simulink library "libGainScheduleDataLoader"  (R2020b)
settings: Solver=VariableStepAuto  StartTime=0.0  StopTime=10.0  RelTol=1e-3
undefined symbols (not defined in the file): range, scheduleData
settings Model: Creator=caatay  LastModifiedBy=caatay

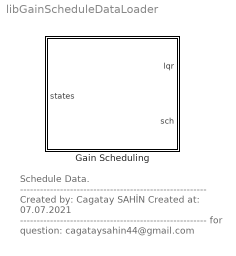
== system libGainScheduleDataLoader ==
  note: Schedule Data.
      | --------------------------------------------------------
      | Created by: Cagatay SAHİN
      | Created at: 07.07.2021
      | --------------------------------------------------------
      | for question:
      | cagataysahin44@gmail.com
  Gain Scheduling : Subsystem  mask(Flight Control System - Gain Scheduling Model - Scheduled Data Loader){scheduleData=scheduleData, range=range}
      mask prompts: scheduleData "Scheduling Data For FCS"; range "Scheduling Data Range"
      mask help: Aircraft's Stability Augmented System's schedule and gain data loader model.
      mask Help:
      | This block is used for obtain schedule database for stability augmented system to stabilize aircraft.
      | --------------------------------------------------------------------------------------------------------------------------------------------------
      | Input of the function:
      | 	states: State Information.
      | Output of the function:
      | 	K_{lqr}: LQR Gain Parameters.
      | 	sch: Scheduled Database Parameters.
      | --------------------------------------------------------------------------------------------------------------------------------------------------
      | for question: "cagataysahin44@gmail.com"
      mask Display:
      | port_label('input',1,'states','texmode','on');
      | 
      | port_label('output',1,'K_{lqr}','texmode','on');
      | port_label('output',2,'Sch','texmode','on');

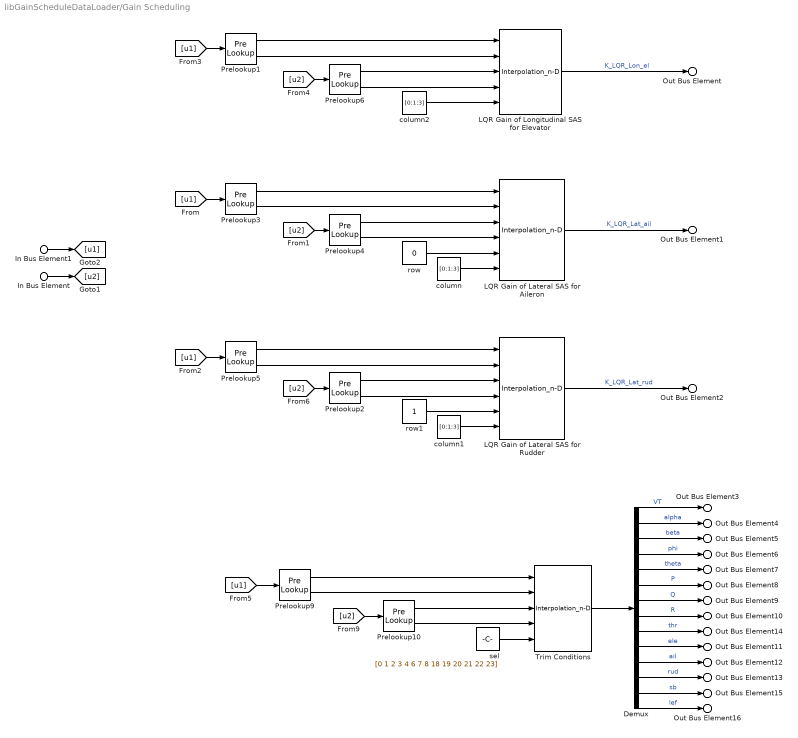
== system libGainScheduleDataLoader/Gain Scheduling ==
  In Bus Element : Inport  PortName=states  Element=tas
  In Bus Element1 : Inport  PortName=states  Element=z_e
  Demux : Demux  Outputs=14
  LQR Gain of Lateral SAS for Aileron : Interpolation_n-D  NumberOfTableDimensions=4  Table=scheduleData.euler.gain.sas.lat  NumSelectionDims=2  InternalRulePriority=Speed
      settings: InputPortMap=u0,u1,u2,u3,u4,u5
  LQR Gain of Lateral SAS for Rudder : Interpolation_n-D  NumberOfTableDimensions=4  Table=scheduleData.euler.gain.sas.lat  NumSelectionDims=2  InternalRulePriority=Speed
      settings: InputPortMap=u0,u1,u2,u3,u4,u5
  LQR Gain of Longitudinal SAS for Elevator : Interpolation_n-D  NumberOfTableDimensions=3  Table=scheduleData.euler.gain.sas.long  NumSelectionDims=1  InternalRulePriority=Speed
      settings: InputPortMap=u0,u1,u2,u3,u4
  Prelookup{1,3,5,9} (4 alike) : PreLookup  BreakpointsData=range.z_e.min:range.z_e.step:range.z_e.max  ExtrapMethod=Linear
  Prelookup{2,4,6,10} (4 alike) : PreLookup  BreakpointsData=range.tas.min:range.tas.step:range.tas.max  ExtrapMethod=Linear
  Trim Conditions : Interpolation_n-D  NumberOfTableDimensions=3  Table=scheduleData.euler.trim  NumSelectionDims=1  InternalRulePriority=Speed
      settings: InputPortMap=u0,u1,u2,u3,u4
  column : Constant  Value=[0:1:3]
  column1 : Constant  Value=[0:1:3]
  column2 : Constant  Value=[0:1:3]
  row : Constant  Value=0
  row1 : Constant
  sel : Constant  Value=[0 1 2 3 4 6 7 8 18 19 20 21 22 23]  VectorParams1D=off
  Out Bus Element : Outport  VectorParamsAs1DForOutWhenUnconnected=off  PortName=lqr  Element=lon_ele
  Out Bus Element1 : Outport  VectorParamsAs1DForOutWhenUnconnected=off  PortName=lqr  Element=lat_ail
  Out Bus Element2 : Outport  VectorParamsAs1DForOutWhenUnconnected=off  PortName=lqr  Element=lat_rud
  Out Bus Element3 : Outport  Port=2  VectorParamsAs1DForOutWhenUnconnected=off  PortName=sch  Element=tas
  Out Bus Element4 : Outport  Port=2  VectorParamsAs1DForOutWhenUnconnected=off  PortName=sch  Element=alpha
  Out Bus Element5 : Outport  Port=2  VectorParamsAs1DForOutWhenUnconnected=off  PortName=sch  Element=beta
  Out Bus Element6 : Outport  Port=2  VectorParamsAs1DForOutWhenUnconnected=off  PortName=sch  Element=phi
  Out Bus Element7 : Outport  Port=2  VectorParamsAs1DForOutWhenUnconnected=off  PortName=sch  Element=theta
  Out Bus Element8 : Outport  Port=2  VectorParamsAs1DForOutWhenUnconnected=off  PortName=sch  Element=p
  Out Bus Element9 : Outport  Port=2  VectorParamsAs1DForOutWhenUnconnected=off  PortName=sch  Element=q
  Out Bus Element10 : Outport  Port=2  VectorParamsAs1DForOutWhenUnconnected=off  PortName=sch  Element=r
  Out Bus Element14 : Outport  Port=2  VectorParamsAs1DForOutWhenUnconnected=off  PortName=sch  Element=thr
  Out Bus Element11 : Outport  Port=2  VectorParamsAs1DForOutWhenUnconnected=off  PortName=sch  Element=ele
  Out Bus Element12 : Outport  Port=2  VectorParamsAs1DForOutWhenUnconnected=off  PortName=sch  Element=ail
  Out Bus Element13 : Outport  Port=2  VectorParamsAs1DForOutWhenUnconnected=off  PortName=sch  Element=rud
  Out Bus Element15 : Outport  Port=2  VectorParamsAs1DForOutWhenUnconnected=off  PortName=sch  Element=sb
  Out Bus Element16 : Outport  Port=2  VectorParamsAs1DForOutWhenUnconnected=off  PortName=sch  Element=lef
  wires:
  Demux/14 -> Out Bus Element16/1  "lef"
  Demux/13 -> Out Bus Element15/1  "sb"
  Demux/9 -> Out Bus Element14/1  "thr"
  Demux/12 -> Out Bus Element13/1  "rud"
  Demux/10 -> Out Bus Element11/1  "ele"
  Demux/11 -> Out Bus Element12/1  "ail"
  Prelookup1/2 -> LQR Gain of Longitudinal SAS for Elevator/2
  LQR Gain of Lateral SAS for Rudder/1 -> Out Bus Element2/1  "K_LQR_Lat_rud"
  Demux/7 -> Out Bus Element9/1  "Q"
  Demux/6 -> Out Bus Element8/1  "P"
  sel/1 -> Trim Conditions/5
  Demux/4 -> Out Bus Element6/1  "phi"
  Prelookup3/2 -> LQR Gain of Lateral SAS for Aileron/2
  [u1] -> Prelookup9/1
  Prelookup4/2 -> LQR Gain of Lateral SAS for Aileron/4
  Prelookup4/1 -> LQR Gain of Lateral SAS for Aileron/3
  Demux/2 -> Out Bus Element4/1  "alpha"
  [u2] -> Prelookup4/1
  Prelookup1/1 -> LQR Gain of Longitudinal SAS for Elevator/1
  column2/1 -> LQR Gain of Longitudinal SAS for Elevator/5
  Prelookup5/1 -> LQR Gain of Lateral SAS for Rudder/1
  [u2] -> Prelookup6/1
  Prelookup9/1 -> Trim Conditions/1
  [u2] -> Prelookup10/1
  column1/1 -> LQR Gain of Lateral SAS for Rudder/6
  column/1 -> LQR Gain of Lateral SAS for Aileron/6
  Prelookup9/2 -> Trim Conditions/2
  LQR Gain of Lateral SAS for Aileron/1 -> Out Bus Element1/1  "K_LQR_Lat_ail"
  Demux/3 -> Out Bus Element5/1  "beta"
  Prelookup3/1 -> LQR Gain of Lateral SAS for Aileron/1
  Prelookup5/2 -> LQR Gain of Lateral SAS for Rudder/2
  [u1] -> Prelookup3/1
  row/1 -> LQR Gain of Lateral SAS for Aileron/5
  Prelookup6/2 -> LQR Gain of Longitudinal SAS for Elevator/4
  Prelookup10/2 -> Trim Conditions/4
  Demux/1 -> Out Bus Element3/1  "VT"
  LQR Gain of Longitudinal SAS for Elevator/1 -> Out Bus Element/1  "K_LQR_Lon_el"
  row1/1 -> LQR Gain of Lateral SAS for Rudder/5
  Demux/5 -> Out Bus Element7/1  "theta"
  [u1] -> Prelookup5/1
  [u1] -> Prelookup1/1
  Prelookup2/2 -> LQR Gain of Lateral SAS for Rudder/4
  [u2] -> Prelookup2/1
  Demux/8 -> Out Bus Element10/1  "R"
  Prelookup6/1 -> LQR Gain of Longitudinal SAS for Elevator/3
  In Bus Element1/1 -> [u1]
  Prelookup2/1 -> LQR Gain of Lateral SAS for Rudder/3
  Trim Conditions/1 -> Demux/1
  Prelookup10/1 -> Trim Conditions/3
  In Bus Element/1 -> [u2]
